simulink model "SimulinkBlockCollection"  (R2023b)
settings: Solver=VariableStepAuto  StartTime=0.0  StopTime=10.0  RelTol=1e-3
undefined symbols (not defined in the file): alpha1, c_D_delta_E, c_D_i, e0_0, e1_0, e2_0, e3_0, eul_0, FTx, fTx, FTy, fTy, FTz, fTz, g, i_H, LT, lT, Mach, mass, MT, mT, NT, nT, pm_0, q0, qbar1, S_ft2, t_max, Vm_0, Weight, xme_0
libraries: shared6dofsys x4, shared6dof x4, sharedtransform x3, sharedutil x1
settings Model: Creator=Owner  LastModifiedBy=Owner

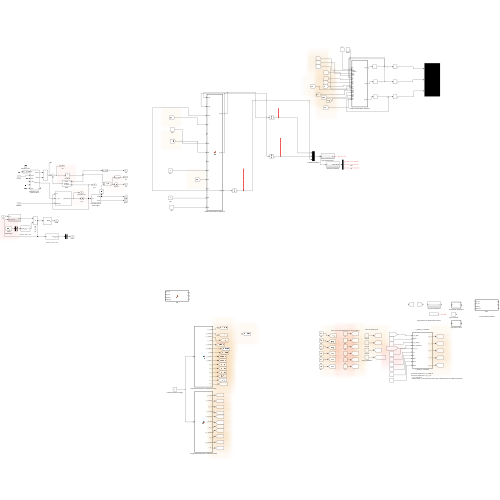
[thumbnail: Simulink's stored preview of the top-level diagram]
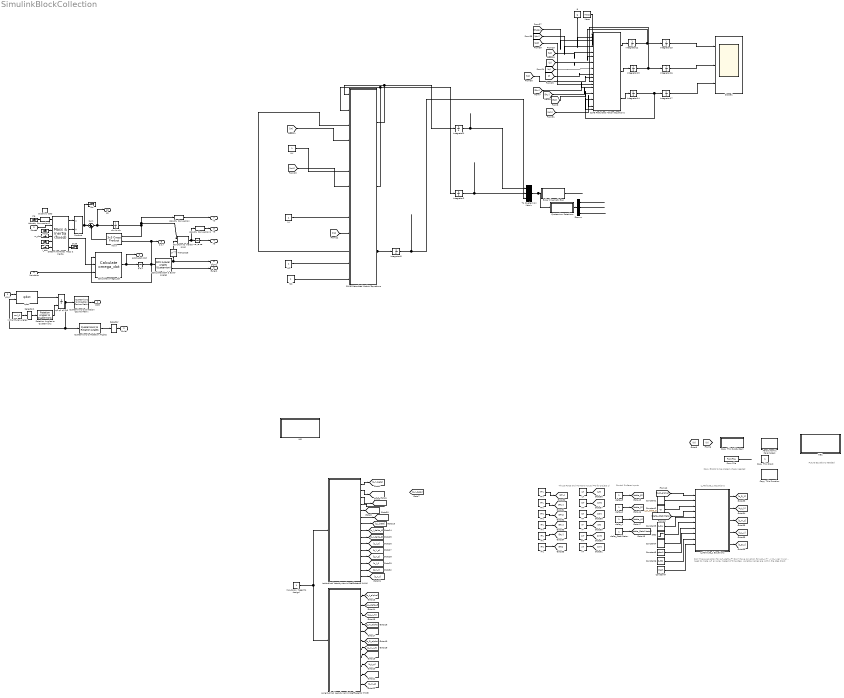
== system SimulinkBlockCollection ==
  note: c_Attribute_1 Equations
  note: Don't have equation for c_D_delta_E?
      | Don't have equation for c_D_i_H?
      | - c_D_i was given
      | - need to make i_H an array based of time step. variable names are within the step block
  note: Thrust Force and Moment Inputs (=0 for project 1)
  note: Control Surface Inputs
  note: Future Equations Needed
  note: Copy Blocks to be placed where needed
  p q r : Inport  OutDataTypeStr=double
  Forces : Inport  Port=2  OutDataTypeStr=double  Unit=lb  PortDimensions=3
  Moments : Inport  Port=3  OutDataTypeStr=double  Unit=lb*ft  PortDimensions=3
  Abi : Terminator
  Aerodynamic Paramaters : MATLAB Function  TreatAsAtomicUnit=on
  CAME Perturbed Motion Equations : MATLAB Function  TreatAsAtomicUnit=on
  CLME Perturbed Motion Equations : MATLAB Function  TreatAsAtomicUnit=on
  Calculate DCM & Euler Angles : shared6dofsys/DCM & Euler Angles (Quaternion)  aMode=aMode
  Calculate omega_dot : shared6dofsys/Calculate omega_dot  aMode=aMode
  Constant1 : Constant  Value=alpha1
  Constant2 : Constant  Value=c_D_delta_E
  Constant3 : Constant  Value=c_D_i
  Constant4 : Constant  Value=Weight
  Constant5 : Constant  Value=qbar1
  Constant6 : Constant  Value=S_ft2
  Constant7 : Constant  Value=Mach
  Copy This Function : MATLAB Function  TreatAsAtomicUnit=on
  Copy This SubSystem : Subsystem
  Copy This block : Constant
  Demux : Demux  Outputs=3
  "Determine Force, Mass & Inertia" : shared6dofsys/Mass & Inertia (fixed)  aMode=aMode
  Disallow CGS : UnitConfiguration  UnitSystemsStr=English,SI,SI (extended)  AllowAllUnitSystems=off
  Euler Kinematic Eqs : Subsystem
  FTx : Constant  Value=FTx
  FTy : Constant  Value=FTy
  FTz : Constant  Value=FTz
  From File : FromFile  SampleTime=0
  From6 : From
  Goto9 : Goto
  I : Ground
  IKE : MATLAB Function  TreatAsAtomicUnit=on
  IKE1 : MATLAB Function  TreatAsAtomicUnit=on
  "IXX " : Constant
  IXZ : Constant
  IYY : Constant
  IZZ : Constant
  I_dot : Ground
  Initial Euler Angles : Constant  Value=eul_0
  InputArray (Need to Assign) : Constant
  Integrator{1..3,12..17} (9 alike) : Integrator
  LT : Constant  Value=LT
  "Latitudinal Aerodynamic Coeffiecents (HW4) " : MATLAB Function  TreatAsAtomicUnit=on
  Longitudinal Aerodynamic Coeffiecents (HW3) : MATLAB Function  TreatAsAtomicUnit=on
  MT : Constant  Value=MT
  Mass : Constant  Value=mass
  NT : Constant  Value=NT
  Out9 : Terminator
  Product : Product  Inputs=*/  SaturateOnIntegerOverflow=on  OutDataTypeStr=Inherit: Same as first input
  Quaternion Rotations : Subsystem
  Quaternions to Direction Cosine Matrix : sharedtransform/Quaternions to  Direction Cosine Matrix  aMode=aMode
  Quaternions to Rotation Angles : sharedtransform/Quaternions to Rotation Angles  rotationOrder=ZYX  aMode=aMode
  Rotation Angles to Quaternions : sharedtransform/Rotation Angles to Quaternions  rotationOrder=ZYX  aMode=aMode
  Scope1 : Scope  NumInputPorts=3
  Selector : Selector  InputPortWidth=3  IndexOptions=Index vector (dialog)  Indices=[3 2 1]  OutputSizes=1
  Selector1 : Selector  InputPortWidth=3  IndexOptions=Index vector (dialog)  Indices=[3 2 1]  OutputSizes=1
  Step : Step  Time=t  Before=i_H  After=t_max  SampleTime=0
  Sum : Sum  Inputs=|++  SaturateOnIntegerOverflow=on
  To Quaternion Matrix : Mux  Inputs=3
  Transpose : Math  Operator=transpose  SignedPower=on
  Vbxw : sharedutil/3x3 Cross Product  aMode=aMode
  Velocity Conversion : shared6dof/6DOF (Euler Angles)/Velocity Conversion  SystemSampleTime=-1  VariantActivationTime=update diagram  AllowFlexibleInterface=on  Latency=0  AutoFrameSizeCalculation=off
  Velocity Conversion1 : shared6dof/6DOF (Euler Angles)/Velocity Conversion1  SystemSampleTime=-1  VariantActivationTime=update diagram  AllowFlexibleInterface=on  Latency=0  AutoFrameSizeCalculation=off
  Velocity Conversion2 : shared6dof/6DOF (Euler Angles)/Velocity Conversion2  SystemSampleTime=-1  VariantActivationTime=update diagram  AllowFlexibleInterface=on  Latency=0  AutoFrameSizeCalculation=off
  Vre : Ground
  c_Attribute_1 Equations : MATLAB Function  TreatAsAtomicUnit=on
  delta_A : Constant
  delta_E : Constant
  delta_R : Constant
  delta_Stabilitator : Constant
  fTx : Constant  Value=fTx
  fTy : Constant  Value=fTy
  fTz : Constant  Value=fTz
  g : Constant  Value=g
  lT : Constant  Value=lT
  mT : Constant  Value=mT
  m_dot : Ground
  mass : Ground
  nT : Constant  Value=nT
  "p,q,r " : Integrator  InitialCondition=pm_0  ContinuousStateAttributes=pm_statename
  q0 q1 q2 q3 : Integrator  InitialConditionSource=external  InitialCondition=[e0_0 e1_0 e2_0 e3_0]  ContinuousStateAttributes=quat_statename
  qdot : shared6dofsys/DCM & Euler Angles (Quaternion)/qdot  SystemSampleTime=-1  VariantActivationTime=update diagram  AllowFlexibleInterface=on  Latency=0  AutoFrameSizeCalculation=off
  "transform to Inertial axes " : shared6dof/6DOF (Euler Angles)/transform to Inertial axes   SystemSampleTime=-1  VariantActivationTime=update diagram  AllowFlexibleInterface=on  Latency=0  AutoFrameSizeCalculation=off
  ub,vb,wb : Integrator  InitialCondition=Vm_0  ContinuousStateAttributes=Vm_statename
  xe,ye,ze : Integrator  InitialCondition=xme_0  ContinuousStateAttributes=xme_statename
  DCM : Outport  OutDataTypeStr=double  VectorParamsAs1DForOutWhenUnconnected=off
  Euler : Outport  Port=2  OutDataTypeStr=double  VectorParamsAs1DForOutWhenUnconnected=off
  Ve : Outport  Port=3  OutDataTypeStr=double  Unit=ft/s  VectorParamsAs1DForOutWhenUnconnected=off
  Xe : Outport  Port=4  OutDataTypeStr=double  Unit=ft  VectorParamsAs1DForOutWhenUnconnected=off
  Euler1 : Outport  Port=5  OutDataTypeStr=double  Unit=rad  VectorParamsAs1DForOutWhenUnconnected=off
  DCM1 : Outport  Port=6  OutDataTypeStr=double  Unit=1  VectorParamsAs1DForOutWhenUnconnected=off
  Vb : Outport  Port=7  OutDataTypeStr=double  Unit=ft/s  VectorParamsAs1DForOutWhenUnconnected=off
  p,q,r : Outport  Port=8  OutDataTypeStr=double  Unit=rad/s  VectorParamsAs1DForOutWhenUnconnected=off
  pdot,qdot,rdot : Outport  Port=9  OutDataTypeStr=double  Unit=rad/s^2  VectorParamsAs1DForOutWhenUnconnected=off
  Ab : Outport  Port=10  OutDataTypeStr=double  Unit=ft/s^2  VectorParamsAs1DForOutWhenUnconnected=off
  wires:
  Longitudinal Aerodynamic Coeffiecents (HW3)/7(c_m_i_H) -> [c_m_i_H]
  "Latitudinal Aerodynamic Coeffiecents (HW4) "/9(c_l_delta_R) -> [c_l_delta_R]
  "Latitudinal Aerodynamic Coeffiecents (HW4) "/13(c_l_r) -> [c_l_r]
  "Latitudinal Aerodynamic Coeffiecents (HW4) "/10(c_l_p) -> [c_l_p]
  "Latitudinal Aerodynamic Coeffiecents (HW4) "/4(c_n_beta) -> ?
  Longitudinal Aerodynamic Coeffiecents (HW3)/3(c_L_i_H) -> [c_L_i_H]
  Longitudinal Aerodynamic Coeffiecents (HW3)/1(c_L_alpha) -> [c_L_alpha]
  "Latitudinal Aerodynamic Coeffiecents (HW4) "/7(c_l_beta) -> [c_l_beta]
  "Latitudinal Aerodynamic Coeffiecents (HW4) "/2(c_Y_delta_A) -> [c_Y_delta_A]
  "Latitudinal Aerodynamic Coeffiecents (HW4) "/12(c_n_p) -> [c_n_p]
  "Latitudinal Aerodynamic Coeffiecents (HW4) "/11(c_Y_p) -> [c_Y_p]
  "Latitudinal Aerodynamic Coeffiecents (HW4) "/3(c_Y_delta_R) -> [c_Y_delta_R]
  Longitudinal Aerodynamic Coeffiecents (HW3)/6(c_D_alpha) -> [c_D_alpha]
  Longitudinal Aerodynamic Coeffiecents (HW3)/9(c_L_q) -> [c_L_q]
  "Latitudinal Aerodynamic Coeffiecents (HW4) "/6(c_n_delta_R) -> [c_n_delta_R]
  "Latitudinal Aerodynamic Coeffiecents (HW4) "/14(c_Y_r) -> [c_Y_r]
  "Latitudinal Aerodynamic Coeffiecents (HW4) "/8(c_l_delta_A) -> [c_l_delta_A]
  "Latitudinal Aerodynamic Coeffiecents (HW4) "/15(c_n_r) -> [c_n_r]
  "Latitudinal Aerodynamic Coeffiecents (HW4) "/5(c_n_delta_A) -> [c_n_delta_A]
  "Latitudinal Aerodynamic Coeffiecents (HW4) "/1(c_Y_beta) -> [c_Y_beta]
  Longitudinal Aerodynamic Coeffiecents (HW3)/11(c_m_q) -> [c_m_q]
  InputArray (Need to Assign)/1 -> Longitudinal Aerodynamic Coeffiecents (HW3)/1(u), "Latitudinal Aerodynamic Coeffiecents (HW4) "/1(u)
  Longitudinal Aerodynamic Coeffiecents (HW3)/2(c_L_delta_E) -> [c_L_delta_E]
  Longitudinal Aerodynamic Coeffiecents (HW3)/8(c_L_alphadot) -> [c_L_alphadot]
  Longitudinal Aerodynamic Coeffiecents (HW3)/10(c_m_alphadot) -> [c_m_alphadot]
  Longitudinal Aerodynamic Coeffiecents (HW3)/5(c_m_delta_E) -> [c_m_delta_E]
  Longitudinal Aerodynamic Coeffiecents (HW3)/4(c_m_alpha) -> [c_m_alpha]
  Demux/2 -> ?  "theta"
  To Quaternion Matrix/1 -> Quaternion Rotations/1(In1), Euler Kinematic Eqs/1(In1)
  Demux/3 -> ?  "psi"
  [p] -> CLME Perturbed Motion Equations/10(p)
  [theta] -> CLME Perturbed Motion Equations/3(theta)
  [V1] -> CLME Perturbed Motion Equations/15(V1)
  IXZ/1 -> CAME Perturbed Motion Equations/12(IXZ)
  CLME Perturbed Motion Equations/2(v_dot) -> Integrator13/1
  [fAy] -> CLME Perturbed Motion Equations/20(fAy)
  [W1] -> CLME Perturbed Motion Equations/24(W1)
  Mass/1 -> CLME Perturbed Motion Equations/1(m)
  [phi] -> CLME Perturbed Motion Equations/5(phi)
  Euler Kinematic Eqs/1(Phi) -> ?
  [fAx] -> CLME Perturbed Motion Equations/18(fAx)
  [U1] -> CLME Perturbed Motion Equations/7(U1)
  IYY/1 -> CAME Perturbed Motion Equations/9(IYY)
  [mA] -> CAME Perturbed Motion Equations/7(mA)
  "IXX "/1 -> CAME Perturbed Motion Equations/6(IXX)
  [lA] -> CAME Perturbed Motion Equations/4(lA)
  Quaternion Rotations/1(Euler Angles) -> Demux/1
  [nA] -> CAME Perturbed Motion Equations/10(nA)
  IZZ/1 -> CAME Perturbed Motion Equations/13(IZZ)
  CAME Perturbed Motion Equations/1(p_dot) -> CAME Perturbed Motion Equations/1("p_dot "), Integrator1/1
  Integrator1/1 -> To Quaternion Matrix/1  "p"
  Integrator2/1 -> To Quaternion Matrix/2  "q"
  [psi] -> CLME Perturbed Motion Equations/17(psi)
  CAME Perturbed Motion Equations/3(r_dot) -> Integrator3/1, CAME Perturbed Motion Equations/3("r_dot ")
  Integrator17/1 -> Scope1/3  "z"
  CAME Perturbed Motion Equations/2(q_dot) -> CAME Perturbed Motion Equations/2("q_dot "), Integrator2/1
  Integrator3/1 -> To Quaternion Matrix/3  "r"
  [fAz] -> CLME Perturbed Motion Equations/22(fAz)
  Integrator13/1 -> CLME Perturbed Motion Equations/16(v), Integrator16/1  "v"
  g/1 -> CLME Perturbed Motion Equations/2(g)
  Integrator14/1 -> CLME Perturbed Motion Equations/25(w), Integrator17/1  "w"
  Demux/1 -> ?
  CLME Perturbed Motion Equations/1(u_dot) -> Integrator12/1
  [q] -> CLME Perturbed Motion Equations/12(q)
  Integrator12/1 -> CLME Perturbed Motion Equations/8(u), Integrator15/1  "u"
  Integrator16/1 -> Scope1/2  "y"
  CLME Perturbed Motion Equations/3(w_dot) -> Integrator14/1
  Integrator15/1 -> Scope1/1  "x"
  [r] -> CLME Perturbed Motion Equations/14(r)
  From File/1 -> ?
  Constant5/1 -> c_Attribute_1 Equations/8(qbar1)
  MT/1 -> [MT]
  Constant3/1 -> c_Attribute_1 Equations/5(c_D_i_H)
  c_Attribute_1 Equations/2(c_L_1) -> [c_L_1]
  FTx/1 -> [FTx]
  lT/1 -> [lT]
  mT/1 -> [mT]
  FTy/1 -> [FTy]
  delta_A/1 -> [delta_A]
  c_Attribute_1 Equations/4(c_L_u) -> [c_L_u]
  Step/1 -> c_Attribute_1 Equations/6(i_H)
  Constant6/1 -> c_Attribute_1 Equations/9(S_ft2)
  Constant4/1 -> c_Attribute_1 Equations/7(W)
  c_Attribute_1 Equations/1(c_D_1) -> [c_D_1]
  LT/1 -> [LT]
  fTx/1 -> [fTx]
  Constant2/1 -> c_Attribute_1 Equations/3(c_D_delta_E)
  c_Attribute_1 Equations/3(c_m_1) -> [c_m_1]
  Constant7/1 -> c_Attribute_1 Equations/10(Mach)
  c_Attribute_1 Equations/5(c_D_u) -> [c_D_u]
  [delta_Stabilitator] -> c_Attribute_1 Equations/4(delta_stabilitator)
  delta_R/1 -> [delta_R]
  NT/1 -> [NT]
  nT/1 -> [nT]
  delta_Stabilitator/1 -> [delta_Stabilitator]
  fTz/1 -> [fTz]
  fTy/1 -> [fTy]
  Constant1/1 -> c_Attribute_1 Equations/2(alpha1)
  FTz/1 -> [FTz]
  [c_D_alpha] -> c_Attribute_1 Equations/1(c_D_alpha)
  delta_E/1 -> [delta_E]
  q0 q1 q2 q3/1 -> qdot/2, Quaternions to Rotation Angles/1, Quaternions to Direction Cosine Matrix/1
  p q r/1 -> qdot/1
  Quaternions to Rotation Angles/1 -> Selector/1
  qdot/1 -> q0 q1 q2 q3/1
  Selector1/1 -> Rotation Angles to Quaternions/1
  Quaternions to Direction Cosine Matrix/1 -> DCM/1
  Initial Euler Angles/1 -> Selector1/1
  Rotation Angles to Quaternions/1 -> q0 q1 q2 q3/2
  Selector/1 -> Euler/1
  "Determine Force, Mass & Inertia"/2 -> Product/2
  Forces/1 -> "Determine Force, Mass & Inertia"/2
  "Determine Force, Mass & Inertia"/3 -> Calculate omega_dot/2
  m_dot/1 -> "Determine Force, Mass & Inertia"/4
  ub,vb,wb/1 -> Vbxw/1, Velocity Conversion/1, "transform to Inertial axes "/1
  Transpose/1 -> "transform to Inertial axes "/2
  Vbxw/1 -> Sum/2
  Calculate DCM & Euler Angles/2 -> Euler1/1
  "transform to Inertial axes "/1 -> xe,ye,ze/1, Velocity Conversion1/1
  Calculate omega_dot/1 -> "p,q,r "/1, pdot,qdot,rdot/1
  "p,q,r "/1 -> Calculate DCM & Euler Angles/1, Calculate omega_dot/1, p,q,r/1, Vbxw/2
  "Determine Force, Mass & Inertia"/4 -> Out9/1
  Product/1 -> Sum/1, Abi/1
  Calculate DCM & Euler Angles/1 -> Transpose/1, DCM1/1
  I/1 -> "Determine Force, Mass & Inertia"/5
  mass/1 -> "Determine Force, Mass & Inertia"/3
  Moments/1 -> Calculate omega_dot/3
  Vre/1 -> Velocity Conversion2/1
  I_dot/1 -> "Determine Force, Mass & Inertia"/6
  Velocity Conversion/1 -> Vb/1
  xe,ye,ze/1 -> Xe/1
  Velocity Conversion2/1 -> "Determine Force, Mass & Inertia"/1
  "Determine Force, Mass & Inertia"/1 -> Product/1
  Sum/1 -> Ab/1, ub,vb,wb/1
  Velocity Conversion1/1 -> Ve/1

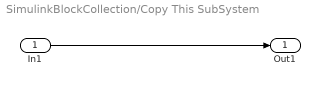
== system SimulinkBlockCollection/Copy This SubSystem ==
  In1 : Inport
  Out1 : Outport
  wires:
  In1/1 -> Out1/1

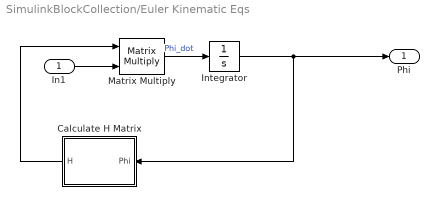
== system SimulinkBlockCollection/Euler Kinematic Eqs ==
  In1 : Inport
  Calculate H Matrix : MATLAB Function  TreatAsAtomicUnit=on
  Integrator : Integrator
  Matrix Multiply : Product  Multiplication=Matrix(*)
  Phi : Outport
  wires:
  In1/1 -> Matrix Multiply/2
  Matrix Multiply/1 -> Integrator/1  "Phi_dot"
  Integrator/1 -> Calculate H Matrix/1(Phi), Phi/1
  Calculate H Matrix/1(H) -> Matrix Multiply/1

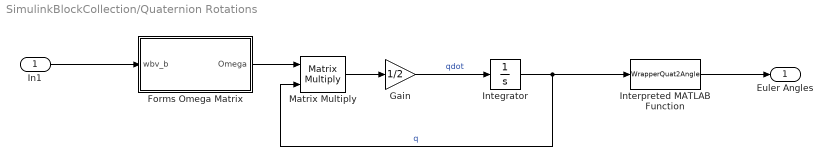
== system SimulinkBlockCollection/Quaternion Rotations ==
  In1 : Inport
  Forms Omega Matrix : MATLAB Function  TreatAsAtomicUnit=on
  Gain : Gain  Gain=1/2
  Integrator : Integrator  InitialCondition=q0
  Interpreted MATLAB Function : MATLABFcn  MATLABFcn=WrapperQuat2Angle
  Matrix Multiply : Product  Multiplication=Matrix(*)
  Euler Angles : Outport
  wires:
  Interpreted MATLAB Function/1 -> Euler Angles/1
  Matrix Multiply/1 -> Gain/1
  Forms Omega Matrix/1(Omega) -> Matrix Multiply/1
  Integrator/1 -> Interpreted MATLAB Function/1, Matrix Multiply/2  "q"
  Gain/1 -> Integrator/1  "qdot"
  In1/1 -> Forms Omega Matrix/1(wbv_b)

== matlab function SimulinkBlockCollection/Longitudinal Aerodynamic Coeffiecents (HW3) ==
  data: u input; c_L_alpha output; c_L_delta_E output; c_L_i_H output; c_m_alpha output; c_m_delta_E output; c_D_alpha output; c_m_i_H output; c_L_alphadot output; c_L_q output; c_m_alphadot output; c_m_q output
function [c_L_alpha, c_L_delta_E, c_L_i_H, c_m_alpha, c_m_delta_E, c_D_alpha, c_m_i_H, c_L_alphadot, c_L_q, c_m_alphadot, c_m_q] = fcn(u)

c_L_alpha_W = c_L_alpha_W_mach;
c_L_alpha_H = c_L_alpha_H_mach*eta_H*(S_H/S_ft2)*(1-d_epsilon_dalpha_mach);
c_L_alpha = c_L_alpha_W_mach + c_L_alpha_H;

c_L_delta_E = 0; 

c_L_i_H = c_L_alpha_H_mach*eta_H*(S_H/S_ft2);

c_m_alpha = (c_L_alpha_W_mach*(xbar_CG - xbar_AC_WB)) - c_L_alpha_H_mach*eta_H*(S_H/S_ft2)*(1-d_epsilon_dalpha_mach)*(xbar_AC_H - xbar_CG);

c_m_i_H = -c_L_alpha_H_mach*eta_H*(S_H/S_ft2) * (xbar_AC_H - xbar_CG);

c_m_delta_E = c_m_i_H * tau_E;

c_D_alpha = ((2*c_L_1)/(pi*AR*e))*c_L_alpha;

c_L_alphadot = 2*c_L_alpha_H_mach*eta_H*(S_H/S_ft2)*(xbar_AC_H - xbar_CG)*(d_epsilon_dalpha_mach);

piece1 = (AR+(2*cos(LambdaLE_quarter_rad)))/(AR*(sqrt((1-Mach^2)*cos(LambdaLE_quarter_rad)^2))+(2*cos(LambdaLE_quarter_rad)));
piece2 = ((0.5+2*abs(xbar_AC_W-xbar_CG))*c_L_alpha_W_mach0);
piece3 = 2*c_L_alpha_H*eta_H*((S_H/S_ft2)*(xbar_AC_H-xbar_CG));
c_L_q = piece1+piece2+piece3;

c_m_alphadot = -2*c_L_alpha_H_mach*eta_H*(S_H/S_ft2)*((xbar_AC_H - xbar_CG)^2)*d_epsilon_dalpha_mach;

lefttopfrac = ((AR^3) * (tan(LambdaLE_quarter_rad)^2))/(AR+(6*cos(LambdaLE_quarter_rad)));
righttopfrac = 3/(sqrt((1-Mach^2)*(cos(LambdaLE_quarter_rad)^2)));
bottomfrac = (((AR^3) * (tan(LambdaLE_quarter_rad)^2))/(AR+(6*(tan(LambdaLE_quarter_rad)^2)))) +3;

secondpiece = -K_q*c_L_alpha_W_mach0*(cos(LambdaLE_quarter_rad));
thirdpiece = ((AR*(0.5*abs(xbar_AC_W-xbar_CG)+(2*abs(xbar_AC_W-xbar_CG)^2)))/(AR+(2*cos(LambdaLEH_quarter_rad)))) + (((1/24) * ((AR^3)* tan(LambdaLE_quarter_rad)^2)/(AR+(6*cos(LambdaLE_quarter_rad))))) + 1/8;
fourthpiece = -2*c_L_alpha_H_mach*eta_H*(S_H/S_ft2)*((xbar_AC_H-xbar_CG)^2) ;
frac = (lefttopfrac+righttopfrac)/(bottomfrac);
c_m_q = (frac * secondpiece * thirdpiece) + fourthpiece;

== matlab function SimulinkBlockCollection/Euler Kinematic Eqs/Calculate H Matrix ==
  data: Phi input; H output
function H = fcn(Phi)

%Unpack Phi
phi     = Phi(1);
theta   = Phi(2);
psi     = Phi(3);

%Input the H matrix
H = [1 tan(theta)*sin(phi) tan(theta)*cos(phi);
    0 cos(phi) -sin(phi);
    0 sin(phi)/cos(theta) cos(phi)/cos(theta)];

== matlab function SimulinkBlockCollection/Quaternion Rotations/Forms Omega Matrix ==
  data: wbv_b input; Omega output
function Omega  = fcn(wbv_b)

wx = wbv_b(1);
wy = wbv_b(2);
wz = wbv_b(3);

Omega = [0 -wx -wy -wz;
    wx 0 wz -wy;
    wy -wz 0 wx;
    wz wy -wx 0];

== matlab function SimulinkBlockCollection/c_Attribute_1 Equations ==
  data: c_D_alpha input; c_D_1 output; alpha1 input; c_D_delta_E input; delta_stabilitator input; c_D_i_H input; i_H input; W input; qbar1 input; S_ft2 input; Mach input; c_L_1 output; c_m_1 output; c_L_u output; c_D_u output
function [c_D_1, c_L_1, c_m_1, c_L_u, c_D_u] = fcn(c_D_alpha, alpha1, c_D_delta_E, delta_stabilitator, c_D_i_H, i_H, W, qbar1, S_ft2, Mach)

c_D_0 = 0;

c_D_1 = c_D_0 + (c_D_alpha*alpha1) + (c_D_delta_E * delta_stabilitator) + (c_D_i_H*i_H);

c_L_1 = W/(qbar1*S_ft2);

c_m_1 = 0;

c_L_u = ((Mach^2)/(1-Mach^2))*c_L_1;

c_D_u = 0;

== matlab function SimulinkBlockCollection/CAME Perturbed Motion Equations ==
  data: p_dot input; p_dot output; q_dot input; r_dot input; lA input; lT input; IXX input; mA input; mT input; IYY input; nA input; nT input; IXZ input; IZZ input; q_dot output; r_dot output
function [p_dot, q_dot, r_dot] = fcn(p_dot, q_dot, r_dot, lA, lT, IXX, mA, mT, IYY, nA, nT, IXZ, IZZ)
%CAME - Still Needs to be fixed
%P_dot = ((la+lt)+(R_dot.*IXZ)+(P.*Q.*IXZ)-((R*Q).*(IZZ-IYY)))./(IXX);
%Q_dot = ((ma+mt)-(R_dot.*IXZ)+(P.*Q.*IXZ)-(R*Q).*(IZZ-IYY))./(IYY);
%R_dot = ((nA+nT) + (P_dot*IXZ) - (((P1*q)+(p*Q1))*(IYY-IXX)) - (((Q1*r)+(R1*q))*IXZ))/(IZZ);

p_dot = ((r_dot*IXZ) + (lA+lT))/IXX;
q_dot = (mA+mT)/IYY;
r_dot = ((nA+nT) + (p_dot*IXZ))/IZZ;

%Need to reorganzie to solve for it

== matlab function SimulinkBlockCollection/IKE ==
  data: phi_dot input; p output; psi_dot input; THETA1 input; theta_dot input; q output; r output
function [p,q,r] = fcn(phi_dot, psi_dot, THETA1, theta_dot)

p = (phi_dot)-(psi_dot*sind(THETA1));
q = theta_dot;
r = psi_dot*cosd(THETA1);


y = u;

== matlab function SimulinkBlockCollection/IKE1 ==
  data: phi_dot input; p output; psi_dot input; THETA1 input; theta_dot input; q output; r output
function [p,q,r] = fcn(phi_dot, psi_dot, THETA1, theta_dot)

p = (phi_dot)-(psi_dot*sind(THETA1));
q = theta_dot;
r = psi_dot*cosd(THETA1);


y = u;

== matlab function SimulinkBlockCollection/Aerodynamic Paramaters ==
  data: u input; y output
function y = fcn(u)

y = u;

== matlab function SimulinkBlockCollection/Copy This Function ==
  data: u input; y output
function y = fcn(u)

y = u;

== matlab function SimulinkBlockCollection/CLME Perturbed Motion Equations ==
  data: m input; u_dot output; g input; theta input; THETA1 input; phi input; PHI1 input; U1 input; u input; P1 input; p input; Q1 input; q input; R1 input; r input; v_dot output; w_dot output; V1 input; v input; psi input; fAx input; fTx input; fAy input; fTy input; fAz input; fTz input; W1 input; w input
function [u_dot, v_dot, w_dot] = fcn(m, g, theta, THETA1, phi, PHI1, U1, u, P1, p, Q1, q, R1, r, V1, v, psi, fAx, fTx, fAy, fTy, fAz, fTz, W1, w)

%Mass = 2300; %kg
%g = 9.81; %m/s
%theta = 0;
%Fax = 0;
%Ftx = 0;

%u_dot = (1/m) * ((-m*g*theta*cosd(THETA1)) + (fAx + fTx) - (Q1*w) - (q*W1) + (R1*v) + (r*V1));
%v_dot = (1/m) * (((-m*g*theta*sind(PHI1)*sind(THETA1))+(m*g*phi*cosd(PHI1)*cosd(THETA1))) + (fAy + fTy) - (U1*r) - (u*R1) + (P1*w) + (p*W1));
%w_dot = (1/m) * (((-m*g*theta*cosd(PHI1)*sind(THETA1))-(m*g*phi*sind(PHI1)*cosd(THETA1))) + (fAz + fTz) - (P1*v) - (V1*p) + (Q1*u) + (U1*q));

u_dot = (1/m) * ((-m*g*theta*cosd(THETA1)) + (fAx + fTx) - (q*W1));
v_dot = (1/m) * ((m*g*phi*cosd(THETA1)) + (fAy+fTy) - (U1*r) + (p*W1));
w_dot = (1/m) * ((-m*g*theta*sind(THETA1)) + (fAz + fTz) + (U1*q));

== matlab function SimulinkBlockCollection/Latitudinal Aerodynamic Coeffiecents (HW4)  ==
  data: u input; c_Y_beta output; c_Y_delta_A output; c_Y_delta_R output; c_n_beta output; c_n_delta_A output; c_n_delta_R output; c_l_beta output; c_l_delta_A output; c_l_delta_R output; c_l_p output; c_Y_p output; c_n_p output; c_l_r output; c_Y_r output; c_n_r output
function [c_Y_beta, c_Y_delta_A, c_Y_delta_R, c_n_beta, c_n_delta_A, c_n_delta_R, c_l_beta, c_l_delta_A, c_l_delta_R, c_l_p, c_Y_p, c_n_p, c_l_r, c_Y_r, c_n_r] = fcn(u)

C_Y_delta_A = 0;

C_Y_delta_R = abs(C_L_alpha_V) *eta_V*((0.5*S2V)/S_ft2)*delta_K_R*tau_R ;

C_Y_beta_W = -.0001 * ((GammaW_deg)) * 57.3 ;
C_Y_beta_H = -.0001 * abs((GammaH_deg)) * 57.3 * (.724 + 3.06 * ((S_H/S_ft2)/(1+cos(rad2deg(LambdaLE_quarter_rad))))+(.4*(ZW_ft/d_ft))+(.009*ARH)) *(S_H/S_ft2);  
C_Y_beta_B = -2*(.96*(SP_V_ft2/S_ft2));
C_Y_beta_V = -K_Y_V * abs(C_L_alpha_V_eff) * (.724 + 3.06 * ((S_V/S_ft2)/(1+cos((LambdaLE_quarter_rad))))+(.4*(ZW_ft/d_ft))+(.009*AR_V_eff)) *(S_V/S_ft2);
C_Y_beta = C_Y_beta_W + C_Y_beta_B + C_Y_beta_H  + C_Y_beta_V ;


y = u;
